simulink library "cstblocks"  (R2025b)
settings: Solver=ode45  StartTime=0.0  StopTime=10.0  RelTol=1e-3
values from neighbouring files (symbols this model uses):
  D = ltipack.lftdataFRD(IC,ltipack.LFTBlockWrapper(blk))    [ControlDesignBlock.m]    (also in DynamicBlock.m = pidstd(ltipack_ssdata(blk)); delayss.m = ltipack.ssdata(a0,b,c,[d0 q;s zeros(length(tau))],[],Ts))
  Ts = blk.Ts_    [DynamicBlock.m]    (also in delayss.m = varargin{1})
undefined symbols (not defined in the file or in its folder): AA, BB, CC, DD, Discrete, INFO, rss, set, Time, uDelay, V, xinit, yDelay
libraries: $bdroot x4, slpidlib x4, cstextras x4, sharedTrackingLibrary x3, ctrlSharedLib x1
(part 3 of 3)

== system cstblocks/Sparse Second Order ==
  In1 : Inport
  DSS : DescriptorStateSpace  E=EE  A=AA  B=BB  C=CC  D=DD  InitialCondition=x0  DirectFeedthrough=Auto  LinearizeToSparse=on
  Out1 : Outport
  wires:
  DSS/1 -> Out1/1
  In1/1 -> DSS/1

== system cstblocks/State Estimation ==
  Extended Kalman Filter : sharedTrackingLibrary/Extended Kalman Filter  StateTransitionFcn=myStateTransitionFcn  HasStateTransitionJacobianFcn=off  HasAdditiveProcessNoise=Additive  ProcessNoise=1  HasTimeVaryingProcessNoise=off  HasStateTransitionFcnExtraArgument=0  InitialState=0  InitialStateCovariance=1  MeasurementFcn1=myMeasurementFcn  HasMeasurementJacobianFcn1=off  HasMeasurementEnablePort1=off  HasAdditiveMeasurementNoise1=Additive  MeasurementNoise1=1  HasTimeVaryingMeasurementNoise1=off  HasMeasurementFcnExtraArgument1=0  HasMeasurementWrapping1=off  MeasurementFcn2=myMeasurementFcn  HasMeasurementJacobianFcn2=off  HasMeasurementEnablePort2=off  HasAdditiveMeasurementNoise2=Additive  MeasurementNoise2=1  HasTimeVaryingMeasurementNoise2=off  HasMeasurementFcnExtraArgument2=0  HasMeasurementWrapping2=off  MeasurementFcn3=myMeasurementFcn  HasMeasurementJacobianFcn3=off  HasMeasurementEnablePort3=off  HasAdditiveMeasurementNoise3=Additive  MeasurementNoise3=1  HasTimeVaryingMeasurementNoise3=off  HasMeasurementFcnExtraArgument3=0  HasMeasurementWrapping3=off  MeasurementFcn4=myMeasurementFcn  HasMeasurementJacobianFcn4=off  HasMeasurementEnablePort4=off  HasAdditiveMeasurementNoise4=Additive  MeasurementNoise4=1  HasTimeVaryingMeasurementNoise4=off  HasMeasurementFcnExtraArgument4=0  HasMeasurementWrapping4=off  MeasurementFcn5=myMeasurementFcn  HasMeasurementJacobianFcn5=off  HasMeasurementEnablePort5=off  HasAdditiveMeasurementNoise5=Additive  MeasurementNoise5=1  HasTimeVaryingMeasurementNoise5=off  HasMeasurementFcnExtraArgument5=0  HasMeasurementWrapping5=off  EnableMultirate=off  StateTransitionFcnSampleTime=1  MeasurementFcn1SampleTime=1  MeasurementFcn2SampleTime=1  MeasurementFcn3SampleTime=1  MeasurementFcn4SampleTime=1  MeasurementFcn5SampleTime=1  UseCurrentEstimator=on  OutputStateCovariance=off  DataType=double  SampleTime=1  NumberOfMeasurements=1
  Kalman Filter : ctrlSharedLib/Kalman Filter  TimeDomain=Discrete-Time  UseCurrentEstimator=on  ModelSource=LTI State-Space Variable  ModelSourceVariable=ss(0.95,1,1,0,1)  A=0.95  B=1  C=1  D=0  NumberOfStates=1  NumberOfInputs=1  NumberOfOutputs=1  InitialEstimateSource=Dialog  X0=0  P0=10  UseK=off  UseGH=off  NumberOfProcessNoiseInputs=1  G=1  TimeInvariantG=on  H=0  TimeInvariantH=on  Q=0.05  TimeInvariantQ=on  R=1  TimeInvariantR=on  N=0  TimeInvariantN=on  AddInputPort=on  AddEnablePort=off  OutputEstimatedY=off  OutputP=off  Ts=-1
  Particle Filter : sharedTrackingLibrary/Particle Filter  StateTransitionFcn=vdpParticleFilterStateFcn  HasStateTransitionFcnExtraArgument=0  NumberOfParticles=1000  InitialDistribution=Gaussian  InitialMean=[0; 0]  InitialCovariance=1  InitialStateBounds=[-3 3; -3 3]  InitialParticles=[]  InitialWeights=[]  CircularVariables=0  StateOrientation=Column  MeasurementLikelihoodFcn1=vdpMeasurementLikelihoodFcn  HasMeasurementEnablePort1=off  HasMeasurementFcnExtraArgument1=0  HasMeasurementEnablePort2=off  HasMeasurementFcnExtraArgument2=0  HasMeasurementEnablePort3=off  HasMeasurementFcnExtraArgument3=0  HasMeasurementEnablePort4=off  HasMeasurementFcnExtraArgument4=0  HasMeasurementEnablePort5=off  HasMeasurementFcnExtraArgument5=0  ResamplingMethod=Multinomial  TriggerMethod=Ratio  MinEffectiveParticleRatio=0.5  SamplingInterval=1  Randomness=Repeatable  Seed=0  StateEstimationMethod=Mean  OutputParticles=off  OutputWeights=off  OutputStateCovariance=off  UseCurrentEstimator=on  EnableMultirate=off  StateTransitionFcnSampleTime=1  MeasurementLikelihoodFcn1SampleTime=1  MeasurementLikelihoodFcn2SampleTime=1  MeasurementLikelihoodFcn3SampleTime=1  MeasurementLikelihoodFcn4SampleTime=1  MeasurementLikelihoodFcn5SampleTime=1  DataType=double  SampleTime=1  NumberOfMeasurements=1
  Unscented Kalman Filter : sharedTrackingLibrary/Unscented Kalman Filter  StateTransitionFcn=myStateTransitionFcn  HasAdditiveProcessNoise=Additive  ProcessNoise=1  HasTimeVaryingProcessNoise=off  HasStateTransitionFcnExtraArgument=0  InitialState=0  InitialStateCovariance=1  Alpha=1e-3  Beta=2  Kappa=0  MeasurementFcn1=myMeasurementFcn  HasMeasurementEnablePort1=off  HasAdditiveMeasurementNoise1=Additive  MeasurementNoise1=1  HasTimeVaryingMeasurementNoise1=off  HasMeasurementFcnExtraArgument1=0  HasMeasurementWrapping1=off  MeasurementFcn2=myMeasurementFcn  HasMeasurementEnablePort2=off  HasAdditiveMeasurementNoise2=Additive  MeasurementNoise2=1  HasTimeVaryingMeasurementNoise2=off  HasMeasurementFcnExtraArgument2=0  HasMeasurementWrapping2=off  MeasurementFcn3=myMeasurementFcn  HasMeasurementEnablePort3=off  HasAdditiveMeasurementNoise3=Additive  MeasurementNoise3=1  HasTimeVaryingMeasurementNoise3=off  HasMeasurementFcnExtraArgument3=0  HasMeasurementWrapping3=off  MeasurementFcn4=myMeasurementFcn  HasMeasurementEnablePort4=off  HasAdditiveMeasurementNoise4=Additive  MeasurementNoise4=1  HasTimeVaryingMeasurementNoise4=off  HasMeasurementFcnExtraArgument4=0  HasMeasurementWrapping4=off  MeasurementFcn5=myMeasurementFcn  HasMeasurementEnablePort5=off  HasAdditiveMeasurementNoise5=Additive  MeasurementNoise5=1  HasTimeVaryingMeasurementNoise5=off  HasMeasurementFcnExtraArgument5=0  HasMeasurementWrapping5=off  EnableMultirate=off  StateTransitionFcnSampleTime=1  MeasurementFcn1SampleTime=1  MeasurementFcn2SampleTime=1  MeasurementFcn3SampleTime=1  MeasurementFcn4SampleTime=1  MeasurementFcn5SampleTime=1  UseCurrentEstimator=on  OutputStateCovariance=off  DataType=double  SampleTime=1  NumberOfMeasurements=1

== system cstblocks/Linear Parameter Varying/Discrete Varying Delay ==
  Inport : Inport  SampleTime=Ts
  TdPort : Inport  Port=2  SampleTime=Ts
  Delay : Delay  DelayLengthSource=Input port  DelayLength=Td  DelayLengthUpperLimit=TdMax  InitialCondition=u0  SampleTime=Ts
      settings: InputPortMap=u0,p1
  Round : Rounding  Operator=round
  TdSat : Saturate  UpperLimit=Inf  LowerLimit=0
  Outport : Outport  VectorParamsAs1DForOutWhenUnconnected=off
  wires:
  TdPort/1 -> TdSat/1
  TdSat/1 -> Round/1
  Inport/1 -> Delay/1
  Delay/1 -> Outport/1
  Round/1 -> Delay/2

== system cstblocks/Linear Parameter Varying/Discrete Varying Lowpass ==
  u : Inport
  frequency : Inport  Port=2
  FOS : cstextras/DiscreteFirstOrderSection  VariantControl=(default)  Ts=Ts  w0=w0
  y : Outport  VectorParamsAs1DForOutWhenUnconnected=off
  wires:
  u/1 -> FOS/1
  frequency/1 -> FOS/2
  FOS/1 -> y/1

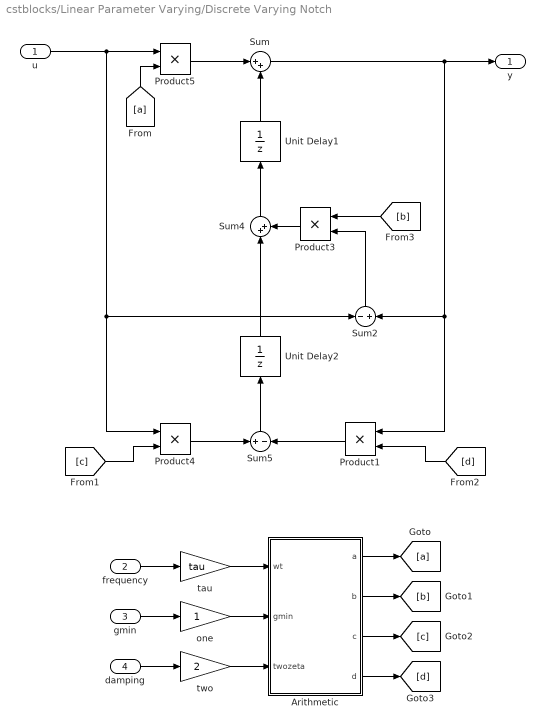
== system cstblocks/Linear Parameter Varying/Discrete Varying Notch ==
  u : Inport
  frequency : Inport  Port=2
  gmin : Inport  Port=3
  damping : Inport  Port=4
  Arithmetic : Subsystem
  Product{1,3..5} (4 alike) : Product
  Sum : Sum  Inputs=|++
  Sum2 : Sum  Inputs=-|+
  Sum4 : Sum  Inputs=|++
  Sum5 : Sum  Inputs=+|-
  Unit Delay1 : UnitDelay  SampleTime=Ts  HasFrameUpgradeWarning=on
  Unit Delay2 : UnitDelay  SampleTime=Ts  HasFrameUpgradeWarning=on
  one : Gain  Tag=#GainSurfaceTarget_
  tau : Gain  Tag=#GainSurfaceTarget_  Gain=tau
  two : Gain  Tag=#GainSurfaceTarget_  Gain=2
  y : Outport  VectorParamsAs1DForOutWhenUnconnected=off
  wires:
  Sum2/1 -> Product3/2
  Sum/1 -> y/1, Sum2/2, Product1/1
  u/1 -> Product4/1, Sum2/1, Product5/1
  Product5/1 -> Sum/1
  Unit Delay1/1 -> Sum/2
  Sum4/1 -> Unit Delay1/1
  Product3/1 -> Sum4/2
  Unit Delay2/1 -> Sum4/1
  Sum5/1 -> Unit Delay2/1
  Product4/1 -> Sum5/1
  Product1/1 -> Sum5/2
  gmin/1 -> one/1
  frequency/1 -> tau/1
  damping/1 -> two/1
  Arithmetic/1(a) -> [a]
  Arithmetic/2(b) -> [b]
  Arithmetic/4(d) -> [d]
  [a] -> Product5/2
  [c] -> Product4/2
  [d] -> Product1/2
  [b] -> Product3/1
  tau/1 -> Arithmetic/1(wt)
  one/1 -> Arithmetic/2(gmin)
  two/1 -> Arithmetic/3(twozeta)
  Arithmetic/3(c) -> [c]

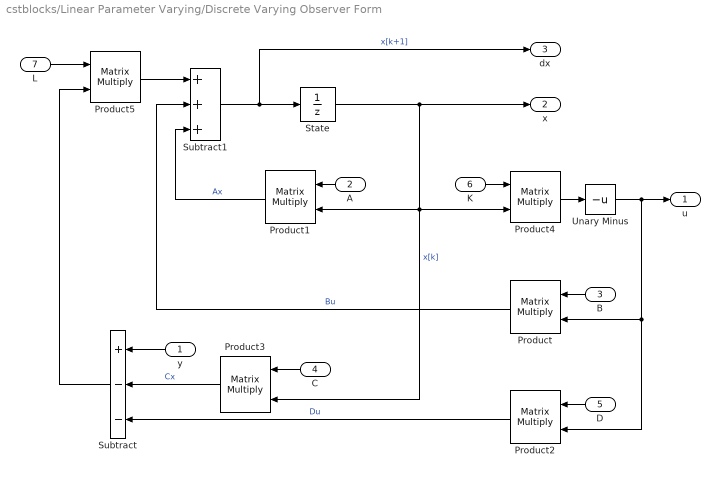
== system cstblocks/Linear Parameter Varying/Discrete Varying Observer Form ==
  y : Inport
  A : Inport  Port=2
  B : Inport  Port=3
  C : Inport  Port=4
  D : Inport  Port=5
  K : Inport  Port=6
  L : Inport  Port=7
  Product{,1..5} (6 alike) : Product  SCDEnableBlockLinearizationSpecification=on  Multiplication=Matrix(*)
  State : UnitDelay  InitialCondition=x0  SampleTime=Ts  HasFrameUpgradeWarning=on
  Subtract : Sum  Inputs=+--
  Subtract1 : Sum  Inputs=+++
  Unary Minus : UnaryMinus
  u : Outport  VectorParamsAs1DForOutWhenUnconnected=off
  x : Outport  Port=2  VectorParamsAs1DForOutWhenUnconnected=off
  dx : Outport  Port=3  VectorParamsAs1DForOutWhenUnconnected=off
  wires:
  Product2/1 -> Subtract/3  "Du"
  Subtract/1 -> Product5/2
  Product3/1 -> Subtract/2  "Cx"
  L/1 -> Product5/1
  Product5/1 -> Subtract1/1
  Product/1 -> Subtract1/2  "Bu"
  y/1 -> Subtract/1
  Unary Minus/1 -> u/1, Product/2, Product2/2
  K/1 -> Product4/1
  Product4/1 -> Unary Minus/1
  Subtract1/1 -> dx/1, State/1  "x[k+1]"
  State/1 -> Product1/2, Product4/2, Product3/2, x/1  "x[k]"
  B/1 -> Product/1
  Product1/1 -> Subtract1/3  "Ax"
  A/1 -> Product1/1
  D/1 -> Product2/1
  C/1 -> Product3/1

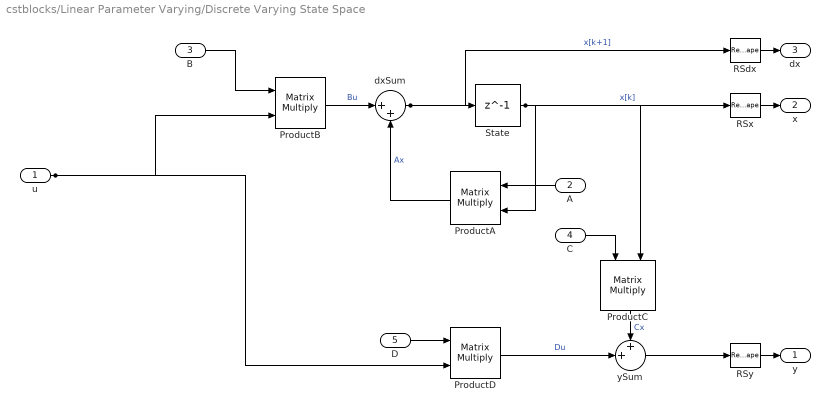
== system cstblocks/Linear Parameter Varying/Discrete Varying State Space ==
  u : Inport  SampleTime=Ts
  A : Inport  Port=2  SampleTime=Ts
  B : Inport  Port=3  SampleTime=Ts
  C : Inport  Port=4  SampleTime=Ts
  D : Inport  Port=5  SampleTime=Ts
  ProductA : Product  SCDEnableBlockLinearizationSpecification=on  Multiplication=Matrix(*)
  ProductB : Product  SCDEnableBlockLinearizationSpecification=on  Multiplication=Matrix(*)
  ProductC : Product  SCDEnableBlockLinearizationSpecification=on  Multiplication=Matrix(*)
  ProductD : Product  SCDEnableBlockLinearizationSpecification=on  Multiplication=Matrix(*)
  RSdx : Reshape
  RSx : Reshape
  RSy : Reshape
  State : Delay  DelayLength=1  InitialCondition=InitialCondition  SampleTime=Ts
  dxSum : Sum  Inputs=|++
  ySum : Sum  Inputs=++|
  y : Outport  VectorParamsAs1DForOutWhenUnconnected=off
  x : Outport  Port=2  VectorParamsAs1DForOutWhenUnconnected=off
  dx : Outport  Port=3  VectorParamsAs1DForOutWhenUnconnected=off
  wires:
  RSy/1 -> y/1
  ySum/1 -> RSy/1
  dxSum/1 -> RSdx/1, State/1  "x[k+1]"
  RSdx/1 -> dx/1
  State/1 -> RSx/1, ProductA/2, ProductC/2  "x[k]"
  RSx/1 -> x/1
  u/1 -> ProductB/2, ProductD/2
  A/1 -> ProductA/1
  B/1 -> ProductB/1
  C/1 -> ProductC/1
  D/1 -> ProductD/1
  ProductB/1 -> dxSum/1  "Bu"
  ProductA/1 -> dxSum/2  "Ax"
  ProductC/1 -> ySum/1  "Cx"
  ProductD/1 -> ySum/2  "Du"

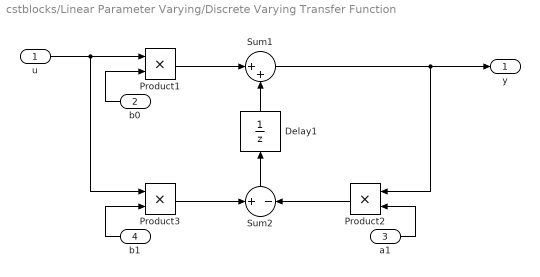
== system cstblocks/Linear Parameter Varying/Discrete Varying Transfer Function ==
  u : Inport
  b0 : Inport  Port=2
  a1 : Inport  Port=3
  b1 : Inport  Port=4
  Delay1 : UnitDelay  SampleTime=Ts  HasFrameUpgradeWarning=on
  Product1 : Product  InputSameDT=on  RndMeth=Zero  SaturateOnIntegerOverflow=on  OutDataTypeStr=Inherit: Same as first input
  Product2 : Product  InputSameDT=on  RndMeth=Zero  SaturateOnIntegerOverflow=on  OutDataTypeStr=Inherit: Same as first input
  Product3 : Product  InputSameDT=on  RndMeth=Zero  SaturateOnIntegerOverflow=on  OutDataTypeStr=Inherit: Same as first input
  Sum1 : Sum  Inputs=|++  InputSameDT=on  SaturateOnIntegerOverflow=on  OutDataTypeStr=Inherit: Same as first input
  Sum2 : Sum  Inputs=+|-  InputSameDT=on  SaturateOnIntegerOverflow=on  OutDataTypeStr=Inherit: Same as first input
  y : Outport  VectorParamsAs1DForOutWhenUnconnected=off
  wires:
  u/1 -> Product1/1, Product3/1
  b0/1 -> Product1/2
  Product1/1 -> Sum1/1
  Sum1/1 -> y/1, Product2/1
  Delay1/1 -> Sum1/2
  Sum2/1 -> Delay1/1
  Product3/1 -> Sum2/1
  Product2/1 -> Sum2/2
  b1/1 -> Product3/2
  a1/1 -> Product2/2

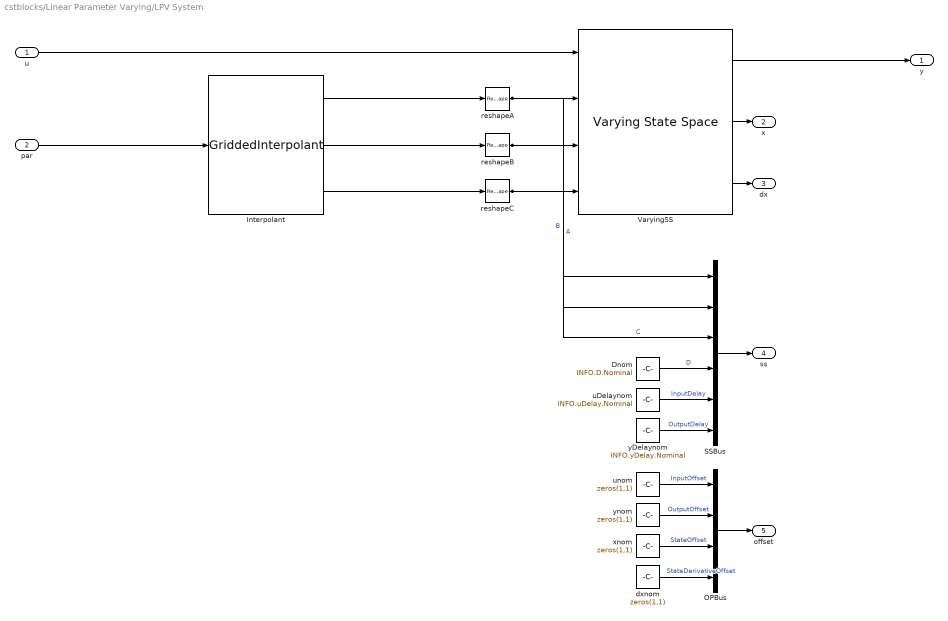
== system cstblocks/Linear Parameter Varying/LPV System ==
  u : Inport  PortDimensions=1
  par : Inport  Port=2  PortDimensions=1
  Dnom : Constant  Value=INFO.D.Nominal  VectorParams1D=off
  Interpolant : cstextras/GriddedInterpolant  Table=V  INFO=INFO  IndexSearch=Binary search  IndexBegin=on
  OPBus : BusCreator  Inputs=4
  SSBus : BusCreator  Inputs=6
  VaryingSS : $bdroot/Linear Parameter Varying/Varying State Space  InitialConditionSource=internal  InitialCondition=InitialCondition  xNames=''  OutputX=on  OutputDX=on  Feedthrough=off  InputX0=off  InputDX0=off  InputU0=off  InputY0=off
  dxnom : Constant  Value=zeros(1,1)  VectorParams1D=off
  reshapeA : Reshape  OutputDimensionality=Customize  OutputDimensions=size(INFO.A.Nominal)
  reshapeB : Reshape  OutputDimensionality=Customize  OutputDimensions=size(INFO.B.Nominal)
  reshapeC : Reshape  OutputDimensionality=Customize  OutputDimensions=size(INFO.C.Nominal)
  uDelaynom : Constant  Value=INFO.uDelay.Nominal  VectorParams1D=off
  unom : Constant  Value=zeros(1,1)  VectorParams1D=off
  xnom : Constant  Value=zeros(1,1)  VectorParams1D=off
  yDelaynom : Constant  Value=INFO.yDelay.Nominal  VectorParams1D=off
  ynom : Constant  Value=zeros(1,1)  VectorParams1D=off
  y : Outport  VectorParamsAs1DForOutWhenUnconnected=off
  x : Outport  Port=2  VectorParamsAs1DForOutWhenUnconnected=off
  dx : Outport  Port=3  VectorParamsAs1DForOutWhenUnconnected=off
  ss : Outport  Port=4  VectorParamsAs1DForOutWhenUnconnected=off
  offset : Outport  Port=5  VectorParamsAs1DForOutWhenUnconnected=off
  wires:
  par/1 -> Interpolant/1
  VaryingSS/2 -> x/1
  VaryingSS/3 -> dx/1
  Interpolant/1 -> reshapeA/1
  reshapeA/1 -> VaryingSS/2, SSBus/1  "A"
  Interpolant/2 -> reshapeB/1
  reshapeB/1 -> VaryingSS/3, SSBus/2  "B"
  Interpolant/3 -> reshapeC/1
  reshapeC/1 -> VaryingSS/4, SSBus/3  "C"
  u/1 -> VaryingSS/1
  VaryingSS/1 -> y/1
  SSBus/1 -> ss/1
  Dnom/1 -> SSBus/4  "D"
  uDelaynom/1 -> SSBus/5  "InputDelay"
  yDelaynom/1 -> SSBus/6  "OutputDelay"
  OPBus/1 -> offset/1
  unom/1 -> OPBus/1  "InputOffset"
  ynom/1 -> OPBus/2  "OutputOffset"
  xnom/1 -> OPBus/3  "StateOffset"
  dxnom/1 -> OPBus/4  "StateDerivativeOffset"

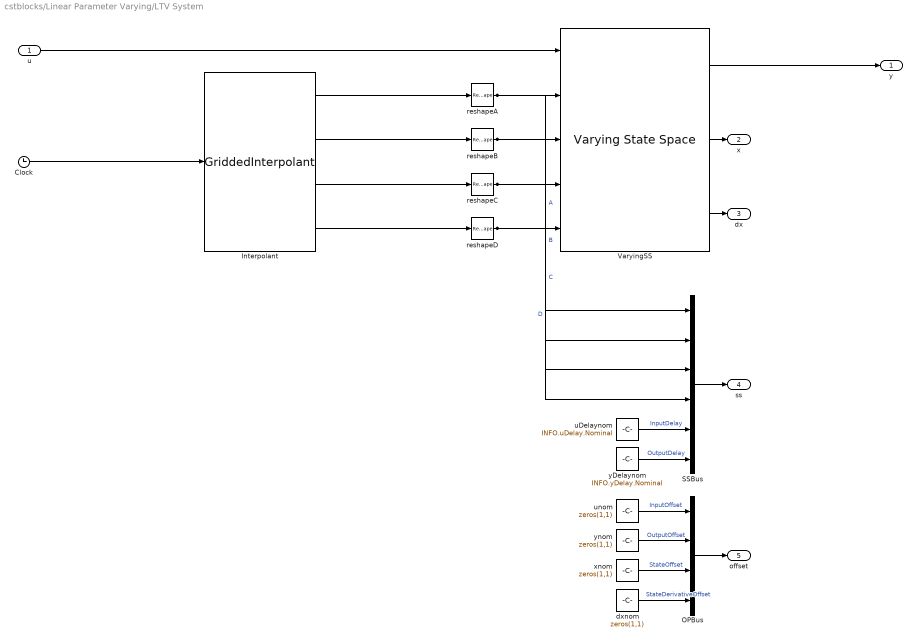
== system cstblocks/Linear Parameter Varying/LTV System ==
  u : Inport  PortDimensions=1
  Clock : Clock
  Interpolant : cstextras/GriddedInterpolant  Table=V  INFO=INFO  IndexSearch=Binary search  IndexBegin=on
  OPBus : BusCreator  Inputs=4
  SSBus : BusCreator  Inputs=6
  VaryingSS : $bdroot/Linear Parameter Varying/Varying State Space  InitialConditionSource=internal  InitialCondition=InitialCondition  xNames=''  OutputX=on  OutputDX=on  Feedthrough=on  InputX0=off  InputDX0=off  InputU0=off  InputY0=off
  dxnom : Constant  Value=zeros(1,1)  VectorParams1D=off
  reshapeA : Reshape  OutputDimensionality=Customize  OutputDimensions=size(INFO.A.Nominal)
  reshapeB : Reshape  OutputDimensionality=Customize  OutputDimensions=size(INFO.B.Nominal)
  reshapeC : Reshape  OutputDimensionality=Customize  OutputDimensions=size(INFO.C.Nominal)
  reshapeD : Reshape  OutputDimensionality=Customize  OutputDimensions=size(INFO.D.Nominal)
  uDelaynom : Constant  Value=INFO.uDelay.Nominal  VectorParams1D=off
  unom : Constant  Value=zeros(1,1)  VectorParams1D=off
  xnom : Constant  Value=zeros(1,1)  VectorParams1D=off
  yDelaynom : Constant  Value=INFO.yDelay.Nominal  VectorParams1D=off
  ynom : Constant  Value=zeros(1,1)  VectorParams1D=off
  y : Outport  VectorParamsAs1DForOutWhenUnconnected=off
  x : Outport  Port=2  VectorParamsAs1DForOutWhenUnconnected=off
  dx : Outport  Port=3  VectorParamsAs1DForOutWhenUnconnected=off
  ss : Outport  Port=4  VectorParamsAs1DForOutWhenUnconnected=off
  offset : Outport  Port=5  VectorParamsAs1DForOutWhenUnconnected=off
  wires:
  Clock/1 -> Interpolant/1
  VaryingSS/2 -> x/1
  VaryingSS/3 -> dx/1
  Interpolant/1 -> reshapeA/1
  reshapeA/1 -> VaryingSS/2, SSBus/1  "A"
  Interpolant/2 -> reshapeB/1
  reshapeB/1 -> VaryingSS/3, SSBus/2  "B"
  Interpolant/3 -> reshapeC/1
  reshapeC/1 -> VaryingSS/4, SSBus/3  "C"
  Interpolant/4 -> reshapeD/1
  reshapeD/1 -> VaryingSS/5, SSBus/4  "D"
  u/1 -> VaryingSS/1
  VaryingSS/1 -> y/1
  SSBus/1 -> ss/1
  uDelaynom/1 -> SSBus/5  "InputDelay"
  yDelaynom/1 -> SSBus/6  "OutputDelay"
  OPBus/1 -> offset/1
  unom/1 -> OPBus/1  "InputOffset"
  ynom/1 -> OPBus/2  "OutputOffset"
  xnom/1 -> OPBus/3  "StateOffset"
  dxnom/1 -> OPBus/4  "StateDerivativeOffset"

== system cstblocks/Linear Parameter Varying/Varying Delay ==
  Inport : Inport
  TdPort : Inport  Port=2
  Delay : VariableTransportDelay  MaximumDelay=TdMax  InitialOutput=u0  MaximumPoints=bufsize  ZeroDelay=on  PadeOrder=PadeOrder
  TdSat : Saturate  UpperLimit=Inf  LowerLimit=TdMin  ZeroCross=off
  Outport : Outport  VectorParamsAs1DForOutWhenUnconnected=off
  wires:
  TdPort/1 -> TdSat/1
  Inport/1 -> Delay/1
  Delay/1 -> Outport/1
  TdSat/1 -> Delay/2

== system cstblocks/Linear Parameter Varying/Varying Lowpass Filter ==
  u : Inport
  frequency : Inport  Port=2
  FOS : cstextras/FirstOrderSection  VariantControl=(default)
  y : Outport  VectorParamsAs1DForOutWhenUnconnected=off
  wires:
  u/1 -> FOS/1
  frequency/1 -> FOS/2
  FOS/1 -> y/1

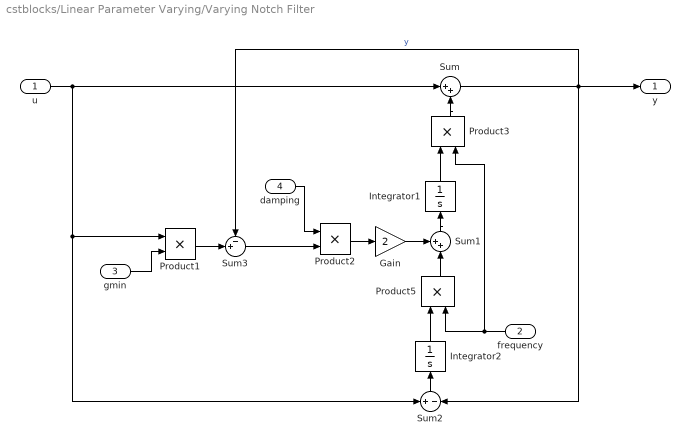
== system cstblocks/Linear Parameter Varying/Varying Notch Filter ==
  u : Inport
  frequency : Inport  Port=2
  gmin : Inport  Port=3
  damping : Inport  Port=4
  Gain : Gain  Gain=2
  Integrator1 : Integrator
  Integrator2 : Integrator
  Product{1..3,5} (4 alike) : Product
  Sum : Sum  Inputs=|++
  Sum1 : Sum  Inputs=++|
  Sum2 : Sum  Inputs=+|-
  Sum3 : Sum  Inputs=-+|
  y : Outport  VectorParamsAs1DForOutWhenUnconnected=off
  wires:
  gmin/1 -> Product1/2
  Sum2/1 -> Integrator2/1
  Product2/1 -> Gain/1
  Sum3/1 -> Product2/2
  Sum/1 -> Sum2/2, y/1, Sum3/1  "y"
  Product1/1 -> Sum3/2
  Sum1/1 -> Integrator1/1
  u/1 -> Sum/1, Product1/1, Sum2/1
  Product3/1 -> Sum/2
  Integrator2/1 -> Product5/1
  frequency/1 -> Product3/2, Product5/2
  Integrator1/1 -> Product3/1
  Product5/1 -> Sum1/2
  Gain/1 -> Sum1/1
  damping/1 -> Product2/1

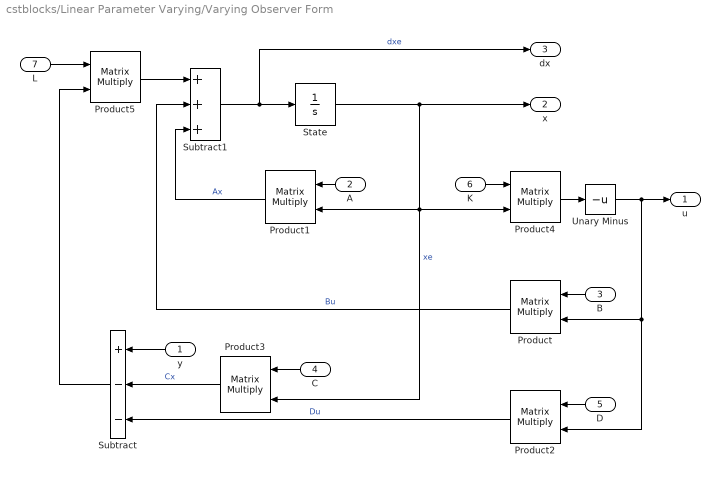
== system cstblocks/Linear Parameter Varying/Varying Observer Form ==
  y : Inport
  A : Inport  Port=2
  B : Inport  Port=3
  C : Inport  Port=4
  D : Inport  Port=5
  K : Inport  Port=6
  L : Inport  Port=7
  Product{,1..5} (6 alike) : Product  SCDEnableBlockLinearizationSpecification=on  Multiplication=Matrix(*)
  State : Integrator  InitialCondition=x0  ContinuousStateAttributes=xNames
  Subtract : Sum  Inputs=+--
  Subtract1 : Sum  Inputs=+++
  Unary Minus : UnaryMinus
  u : Outport  VectorParamsAs1DForOutWhenUnconnected=off
  x : Outport  Port=2  VectorParamsAs1DForOutWhenUnconnected=off
  dx : Outport  Port=3  VectorParamsAs1DForOutWhenUnconnected=off
  wires:
  Product2/1 -> Subtract/3  "Du"
  Subtract/1 -> Product5/2
  Product3/1 -> Subtract/2  "Cx"
  L/1 -> Product5/1
  Product5/1 -> Subtract1/1
  Product/1 -> Subtract1/2  "Bu"
  y/1 -> Subtract/1
  Unary Minus/1 -> u/1, Product/2, Product2/2
  K/1 -> Product4/1
  Product4/1 -> Unary Minus/1
  Subtract1/1 -> dx/1, State/1  "dxe"
  State/1 -> Product1/2, Product4/2, Product3/2, x/1  "xe"
  B/1 -> Product/1
  Product1/1 -> Subtract1/3  "Ax"
  A/1 -> Product1/1
  D/1 -> Product2/1
  C/1 -> Product3/1

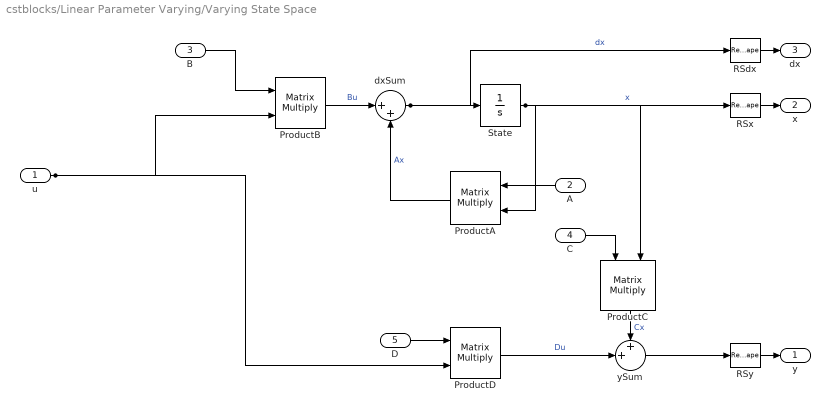
== system cstblocks/Linear Parameter Varying/Varying State Space ==
  u : Inport
  A : Inport  Port=2
  B : Inport  Port=3
  C : Inport  Port=4
  D : Inport  Port=5
  ProductA : Product  SCDEnableBlockLinearizationSpecification=on  Multiplication=Matrix(*)
  ProductB : Product  SCDEnableBlockLinearizationSpecification=on  Multiplication=Matrix(*)
  ProductC : Product  SCDEnableBlockLinearizationSpecification=on  Multiplication=Matrix(*)
  ProductD : Product  SCDEnableBlockLinearizationSpecification=on  Multiplication=Matrix(*)
  RSdx : Reshape
  RSx : Reshape
  RSy : Reshape
  State : Integrator  InitialCondition=InitialCondition  ContinuousStateAttributes=xNames
  dxSum : Sum  Inputs=|++
  ySum : Sum  Inputs=++|
  y : Outport  VectorParamsAs1DForOutWhenUnconnected=off
  x : Outport  Port=2  VectorParamsAs1DForOutWhenUnconnected=off
  dx : Outport  Port=3  VectorParamsAs1DForOutWhenUnconnected=off
  wires:
  RSy/1 -> y/1
  ySum/1 -> RSy/1
  dxSum/1 -> RSdx/1, State/1  "dx"
  RSdx/1 -> dx/1
  State/1 -> RSx/1, ProductA/2, ProductC/2  "x"
  RSx/1 -> x/1
  u/1 -> ProductB/2, ProductD/2
  A/1 -> ProductA/1
  B/1 -> ProductB/1
  C/1 -> ProductC/1
  D/1 -> ProductD/1
  ProductB/1 -> dxSum/1  "Bu"
  ProductA/1 -> dxSum/2  "Ax"
  ProductC/1 -> ySum/1  "Cx"
  ProductD/1 -> ySum/2  "Du"

== system cstblocks/Linear Parameter Varying/Varying Transfer Function ==
  u : Inport
  b0 : Inport  Port=2
  a1 : Inport  Port=3
  b1 : Inport  Port=4
  Integrator1 : Integrator
  Product1 : Product  InputSameDT=on  RndMeth=Zero  SaturateOnIntegerOverflow=on  OutDataTypeStr=Inherit: Same as first input
  Product2 : Product  InputSameDT=on  RndMeth=Zero  SaturateOnIntegerOverflow=on  OutDataTypeStr=Inherit: Same as first input
  Product3 : Product  InputSameDT=on  RndMeth=Zero  SaturateOnIntegerOverflow=on  OutDataTypeStr=Inherit: Same as first input
  Sum1 : Sum  Inputs=|++  InputSameDT=on  SaturateOnIntegerOverflow=on  OutDataTypeStr=Inherit: Same as first input
  Sum2 : Sum  Inputs=+|-  InputSameDT=on  SaturateOnIntegerOverflow=on  OutDataTypeStr=Inherit: Same as first input
  y : Outport  VectorParamsAs1DForOutWhenUnconnected=off
  wires:
  u/1 -> Product1/1, Product3/1
  b0/1 -> Product1/2
  Product1/1 -> Sum1/1
  Sum1/1 -> y/1, Product2/1
  Integrator1/1 -> Sum1/2
  Sum2/1 -> Integrator1/1
  Product3/1 -> Sum2/1
  Product2/1 -> Sum2/2
  b1/1 -> Product3/2
  a1/1 -> Product2/2

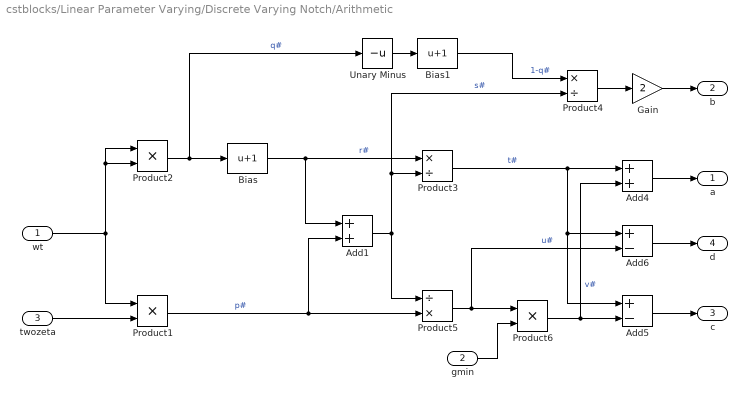
== system cstblocks/Linear Parameter Varying/Discrete Varying Notch/Arithmetic ==
  wt : Inport
  gmin : Inport  Port=2
  twozeta : Inport  Port=3
  Add1 : Sum
  Add4 : Sum
  Add5 : Sum  Inputs=+-
  Add6 : Sum  Inputs=+-
  Bias : Bias  Bias=1  SaturateOnIntegerOverflow=off
  Bias1 : Bias  Bias=1  SaturateOnIntegerOverflow=off
  Gain : Gain  Gain=2
  Product1 : Product
  Product2 : Product
  Product3 : Product  Inputs=*/
  Product4 : Product  Inputs=*/
  Product5 : Product  Inputs=/*
  Product6 : Product
  Unary Minus : UnaryMinus
  a : Outport
  b : Outport  Port=2
  c : Outport  Port=3
  d : Outport  Port=4
  wires:
  Bias1/1 -> Product4/1  "1-q#"
  Add1/1 -> Product5/1, Product3/2, Product4/2  "s#"
  Product1/1 -> Add1/2, Product5/2  "p#"
  Bias/1 -> Product3/1, Add1/1  "r#"
  Product2/1 -> Unary Minus/1, Bias/1  "q#"
  wt/1 -> Product2/1, Product2/2, Product1/1
  twozeta/1 -> Product1/2
  Product4/1 -> Gain/1
  Gain/1 -> b/1
  Product3/1 -> Add5/1, Add6/1, Add4/1  "t#"
  Product5/1 -> Product6/1, Add6/2  "u#"
  gmin/1 -> Product6/2
  Product6/1 -> Add4/2, Add5/2  "v#"
  Add4/1 -> a/1
  Add5/1 -> c/1
  Add6/1 -> d/1
  Unary Minus/1 -> Bias1/1
